simulink model "TUUM1_ME13"  (R2021b)
settings: Solver=ode1  StartTime=0.0  StopTime=Tsim  FixedStep=Ts  RelTol=1e-3
InitFcn:
  | Ts=1e-3;
  | Tsim=14.9;
  | TUUM1;
values from neighbouring files (symbols this model uses):
  REF = 5    [TUUM1.m]
undefined symbols (not defined in the file or in its folder): rtblkgui
libraries: simulink x3
settings Model: SimulationMode=external  Creator=Labos1  LastModifiedBy=Melab1Guest
settings SolverCC: AlgebraicLoopSolver=TrustRegion
settings DataIOCC: ReturnWorkspaceOutputs=off
settings OptimizationCC: LifeSpan=inf
settings DebuggingCC: SFExecutionAtInitializationDiag=none  SFMachineParentedDataDiag=warning  ArithmeticOperatorsInVariantConditions=warning
settings SFSimCC: SimUseLocalCustomCode=off  CustomCodeUndefinedFunction=UseInterfaceOnly
settings RTWCC: Description=Simulink Desktop Real-Time  SystemTargetFile=sldrt.tlc  TemplateMakefile=sldrt.tmf  RTWUseLocalCustomCode=off  RTWCompilerOptimization=on
settings CodeAppCC: MaxIdLength=95  StateflowObjectComments=on
settings SimulinkDesktopRealTimeCC: TargetPreCompLibLocation=C:\Program Files\MATLAB\R2021b\toolbox\sldrt\lib\win64  SupportVariableSizeSignals=off

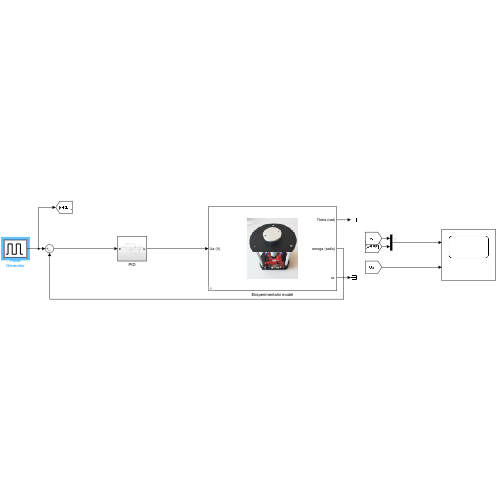
[thumbnail: Simulink's stored preview of the top-level diagram]
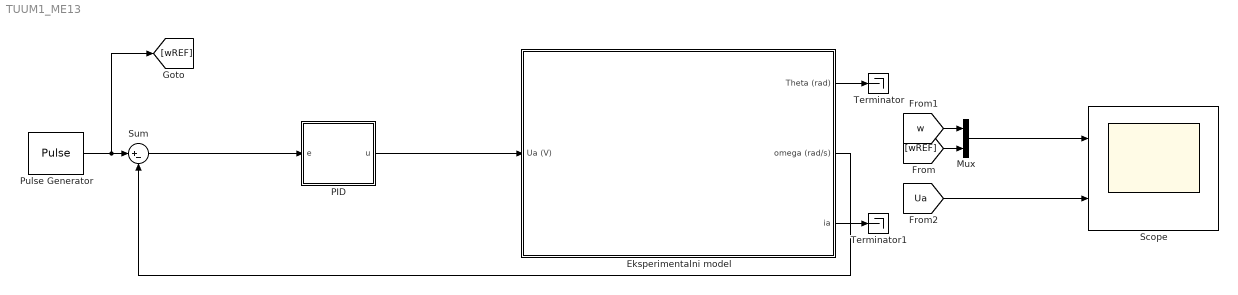
== system TUUM1_ME13 ==
  Eksperimentalni model : Subsystem  mask{R6=383, motorRes=2849.3, Ts=Ts}
      mask init:
      | currentBlock = gcb;
      | %% Closing all the ports:
      | Port = '';
      | FullPort = '';
      | if ~isempty(instrfind)
      |     fclose(instrfind);
      |     delete(instrfind);
      | end
      | %% Find all the COM ports in a computer
      | s1 = instrhwinfo('serial');
      | coms = s1.AvailableSerialPorts;
      | key = 'HKEY_LOCAL_MACHINE\SYSTEM\CurrentControlSet\Enum\USB\';
      | % Find all installed USB devices entries and clean up the output
      | [~, vals] = dos(['REG QUERY ' key ' /s /f "FriendlyName" /t "REG_SZ"']);
      | vals = textscan(vals,'%s','delimiter','\t');
      | vals = cat(1,vals{:});
      | out = 0;
      | % Find all friendly name property entries
      | for i = 1:numel(vals)
      |     if strcmp(vals{i}(1:min(12,end)),'FriendlyName')
      |         if ~iscell(out)
      |             out = vals(i);
      |         else
      |             out{end+1} = vals{i};
      |         end
      |     end
      | end
      | % Compare friendly name entries with connected ports and generate output
      | devs = cell(numel(coms),2);
      | for i = 1:numel(coms)
      |   match = strfind(out,[coms{i},')']);
      |   ind = 0;
      |   for j = 1:numel(match)
      |       if ~isempty(match{j})
      |           ind = j;
      |       end
      |   end
      |   if ind ~= 0
      |       com = str2double(coms{i}(4:end));
      | % Trim the trailing ' (COM##)' from the friendly name - works on ports from 1 to 99
      |       if com > 9
      |           length = 8;
      |       else
      |           length = 7;
      |       end
      |       devs{i,1} = out{ind}(27:end-length);
      |       devs{i,2} = com;
      |   end
      | end
      | % Find USB device
      | for i = size(devs,1)
      |     if strfind(devs{i,1},'USB Serial Device')
      |         ind = i;
      |     end
      | end
      | if ~ind
      |     Port = [];
      | else
      |     port = coms(ind);
      |     Port = port{1};
      | end
      | if (isempty(Port))
      |  %   msgbox('Barbell lab board not found, make sure it is connected, FTDI driver is installed and try again')
      | else
      |     %% Set Packet Input and Packet Output parameters
      |     po = strcat(currentBlock,'/Packet Output1');
      |     pinput = strcat(currentBlock,'/Packet Input1');
      |     %%
      |     set_param(po, 'LinkStatus','inactive');
      |     set_param(pinput, 'LinkStatus','inactive');
      |     %%
      |     p = Simulink.Mask.get(po);
      |     a = p.Parameters(6);
      |     FullPort = Port;
      |     Port = replace(Port,'COM','');
      |     if isempty(Port)
      |         Port = a.Value
      |     end
      |     %%
      | 
      |     a.set('Value',Port);
      |     %%
      |     %%
      |     %%
      |     p1 = Simulink.Mask.get(pinput);
      |     a1 = p1.Parameters(6);
      |     a1.set('Value',Port);
      | 
      | end
      mask Display:
      | ud = get_param(gcb,'UserData');
      | image(ud.x);
  Mux : Mux  Inputs=2
  PID : Subsystem
  Pulse Generator : DiscretePulseGenerator  PulseType=Time based  Amplitude=REF  Period=5  PulseWidth=50
  Scope : Scope  NumInputPorts=2
  Sum : Sum  Inputs=|+-
  Terminator : Terminator
  Terminator1 : Terminator
  wires:
  [w] -> Mux/1
  [wREF] -> Mux/2
  Pulse Generator/1 -> [wREF], Sum/1
  Eksperimentalni model/2(omega (rad/s)) -> Sum/2
  Mux/1 -> Scope/1
  [Ua] -> Scope/2
  Eksperimentalni model/1(Theta (rad)) -> Terminator/1
  Eksperimentalni model/3("ia ") -> Terminator1/1
  Sum/1 -> PID/1(e)
  PID/1(u) -> Eksperimentalni model/1(Ua (V))

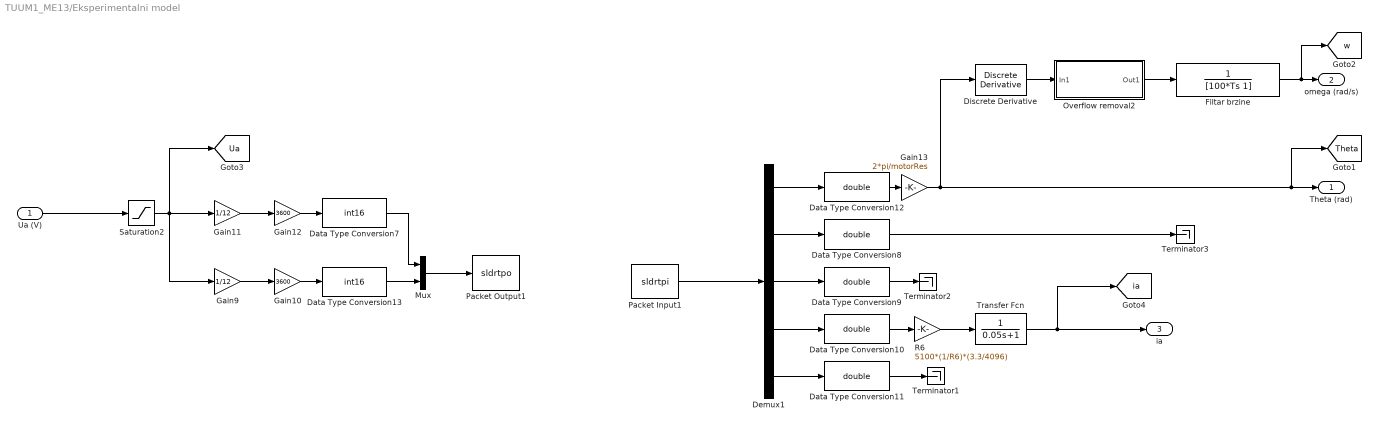
== system TUUM1_ME13/Eksperimentalni model ==
  Ua (V) : Inport
  Data Type Conversion{8..12} (5 alike) : DataTypeConversion  OutDataTypeStr=double
  Data Type Conversion13 : DataTypeConversion  OutDataTypeStr=int16
  Data Type Conversion7 : DataTypeConversion  OutDataTypeStr=int16
  Demux1 : Demux  Outputs=5
  Discrete Derivative : simulink/Discrete/Discrete Derivative  gainval=1.0  ICPrevScaledInput=0.0  OutMin=[]  OutMax=[]  OutDataType=fixdt(1, 16)  OutScaling=2^-10  DoSatur=off
  Filtar brzine : TransferFcn  Denominator=[100*Ts 1]
  Gain10 : Gain  Gain=3600
  Gain11 : Gain  Gain=1/12
  Gain12 : Gain  Gain=3600
  Gain13 : Gain  Gain=2*pi/motorRes  OutDataTypeStr=double
  Gain9 : Gain  Gain=1/12
  Mux : Mux  Inputs=2
  Overflow removal2 : Subsystem
  Packet Input1 : S-Function  LoadFcn=rtblkgui('Load')  StartFcn=rtblkgui('Start',1)  StopFcn=rtblkgui('Start',0)  FunctionName=sldrtpi  Parameters=SampleTime,MaxMissedTicks,ShowMissedTicks,YieldWhenWaiting,DrvName,DrvAddress,DrvOptions,PacketSize,DataTypes,ShowReady,ShowError,PacketID,ByteOrder,ShowTimestamp  SFunctionDeploymentMode=off  EnableBusSupport=off  mask(Simulink Desktop Real-Time Packet Input){SampleTime=Ts, MaxMissedTicks=10, ShowMissedTicks=off, YieldWhenWaiting=off, DrvName=Standard_Devices/Serial_Port, DrvAddress=9, DrvOptions=[115200 8 0 0 0 0 0 0], PacketSize=5*2, DataTypes='5*int16', ShowReady=off, ShowError=off, PacketID=1, ByteOrder=1, ShowTimestamp=off}
      mask prompts: SampleTime "sldrt:sldrtlib:ParamSampleTime"; MaxMissedTicks "sldrt:sldrtlib:ParamMaxMissedTicks"; ShowMissedTicks "sldrt:sldrtlib:ParamShowMissedTicks"; YieldWhenWaiting "sldrt:sldrtlib:ParamYieldWhenWaiting"; DrvName "sldrt:sldrtlib:ParamDriverName"; DrvAddress "sldrt:sldrtlib:ParamDriverAddress"; DrvOptions "sldrt:sldrtlib:ParamDriverOptions"; PacketSize "sldrt:sldrtlib:ParamInputPacketSize"; DataTypes "sldrt:sldrtlib:ParamPacketInputDataTypes"; ShowReady "sldrt:sldrtlib:ParamShowDataReady"; ShowError "sldrt:sldrtlib:ParamShowDataError"; PacketID "sldrt:sldrtlib:ParamPacketIdentifier"; ByteOrder "sldrt:sldrtlib:ParamPacketInputByteOrder"; ShowTimestamp "sldrt:sldrtlib:ParamShowPacketTimestamp"
      mask help: sldrt:sldrtlib:DescPacketInput
      settings: AttributesFormatString=Serial Port [3]  ModelCloseFcn=close(findall(0, 'Type', 'figure', 'Tag', 'SLDRT_RTBLKGUI', 'UserData', gcbh))  OpenFcn=rtblkgui('Open','PI')  ParentCloseFcn=eval(get_param(gcbh, 'ModelCloseFcn'))
      mask Help: helpview(fullfile(docroot, 'toolbox', 'sldrt', 'helptargets.map'), 'rtw_packet_in')
      mask Display: disp('Packet\nInput')
  Packet Output1 : S-Function  LoadFcn=rtblkgui('Load')  StartFcn=rtblkgui('Start',1)  StopFcn=rtblkgui('Start',0)  FunctionName=sldrtpo  Parameters=SampleTime,MaxMissedTicks,ShowMissedTicks,YieldWhenWaiting,DrvName,DrvAddress,DrvOptions,PacketSize,DataTypes,ShowReady,ShowError,PacketID,ByteOrder,InitialValue,FinalValue  SFunctionDeploymentMode=off  EnableBusSupport=off  mask(Simulink Desktop Real-Time Packet Output){SampleTime=Ts, MaxMissedTicks=10, ShowMissedTicks=off, YieldWhenWaiting=off, DrvName=Standard_Devices/Serial_Port, DrvAddress=9, DrvOptions=[115200 8 0 0 0 0 0 0], PacketSize=4, DataTypes='2*int16', ShowReady=off, ShowError=off, PacketID=1, ByteOrder=1, InitialValue=[32767 2], FinalValue=[0 0]}
      mask prompts: SampleTime "sldrt:sldrtlib:ParamSampleTime"; MaxMissedTicks "sldrt:sldrtlib:ParamMaxMissedTicks"; ShowMissedTicks "sldrt:sldrtlib:ParamShowMissedTicks"; YieldWhenWaiting "sldrt:sldrtlib:ParamYieldWhenWaiting"; DrvName "sldrt:sldrtlib:ParamDriverName"; DrvAddress "sldrt:sldrtlib:ParamDriverAddress"; DrvOptions "sldrt:sldrtlib:ParamDriverOptions"; PacketSize "sldrt:sldrtlib:ParamOutputPacketSize"; DataTypes "sldrt:sldrtlib:ParamPacketOutputDataTypes"; ShowReady "sldrt:sldrtlib:ParamShowDataReady"; ShowError "sldrt:sldrtlib:ParamShowDataError"; PacketID "sldrt:sldrtlib:ParamPacketIdentifier"; ByteOrder "sldrt:sldrtlib:ParamPacketOutputByteOrder"; InitialValue "sldrt:sldrtlib:ParamInitialValue"; FinalValue "sldrt:sldrtlib:ParamFinalValue"
      mask help: sldrt:sldrtlib:DescPacketOutput
      settings: AttributesFormatString=Serial Port [3]  ModelCloseFcn=close(findall(0, 'Type', 'figure', 'Tag', 'SLDRT_RTBLKGUI', 'UserData', gcbh))  OpenFcn=rtblkgui('Open','PO')  ParentCloseFcn=eval(get_param(gcbh, 'ModelCloseFcn'))
      mask Help: helpview(fullfile(docroot, 'toolbox', 'sldrt', 'helptargets.map'), 'rtw_packet_out')
      mask Display: disp('Packet\nOutput')
  R6 : Gain  Gain=5100*(1/R6)*(3.3/4096)
  Saturation2 : Saturate  UpperLimit=12  LowerLimit=-12
  Terminator1 : Terminator
  Terminator2 : Terminator
  Terminator3 : Terminator
  Transfer Fcn : TransferFcn  Denominator=[0.05 1]
  Theta (rad) : Outport  VectorParamsAs1DForOutWhenUnconnected=off
  omega (rad/s) : Outport  Port=2  VectorParamsAs1DForOutWhenUnconnected=off
  "ia " : Outport  Port=3  VectorParamsAs1DForOutWhenUnconnected=off
  tag scope: Theta=global, Ua=global, ia=global, w=global
  wires:
  Ua (V)/1 -> Saturation2/1
  Gain12/1 -> Data Type Conversion7/1
  Gain11/1 -> Gain12/1
  Gain10/1 -> Data Type Conversion13/1
  Gain9/1 -> Gain10/1
  Demux1/1 -> Data Type Conversion12/1
  Demux1/2 -> Data Type Conversion8/1
  Demux1/3 -> Data Type Conversion9/1
  Demux1/4 -> Data Type Conversion10/1
  Demux1/5 -> Data Type Conversion11/1
  Saturation2/1 -> [Ua], Gain9/1, Gain11/1
  Data Type Conversion7/1 -> Mux/1
  Data Type Conversion13/1 -> Mux/2
  Data Type Conversion8/1 -> Terminator3/1
  Data Type Conversion12/1 -> Gain13/1
  Gain13/1 -> [Theta], Theta (rad)/1, Discrete Derivative/1
  Discrete Derivative/1 -> Overflow removal2/1(In1)
  Filtar brzine/1 -> [w], omega (rad/s)/1
  Mux/1 -> Packet Output1/1
  Data Type Conversion11/1 -> Terminator1/1
  Data Type Conversion10/1 -> R6/1
  Data Type Conversion9/1 -> Terminator2/1
  R6/1 -> Transfer Fcn/1
  Overflow removal2/1(Out1) -> Filtar brzine/1
  Packet Input1/1 -> Demux1/1
  Transfer Fcn/1 -> [ia], "ia "/1

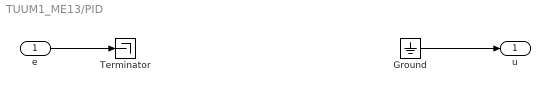
== system TUUM1_ME13/PID ==
  e : Inport
  Ground : Ground
  Terminator : Terminator
  u : Outport
  wires:
  e/1 -> Terminator/1
  Ground/1 -> u/1

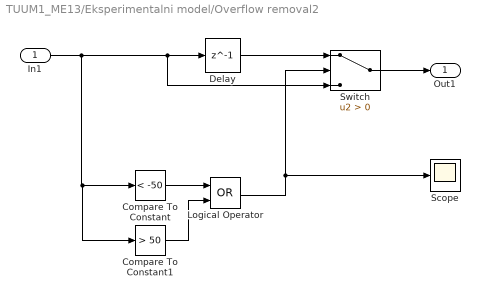
== system TUUM1_ME13/Eksperimentalni model/Overflow removal2 ==
  In1 : Inport
  Compare To Constant : simulink/Logic and Bit Operations/Compare To Constant  relop=<  const=-50  OutDataTypeStr=boolean
  Compare To Constant1 : simulink/Logic and Bit Operations/Compare To Constant  relop=>  const=50  OutDataTypeStr=boolean
  Delay : Delay  DelayLength=1  InitialCondition=0  UseCircularBuffer=on
  Logical Operator : Logic  Operator=OR  AllPortsSameDT=off  OutDataTypeStr=boolean
  Scope : Scope
  Switch : Switch  Criteria=u2 > Threshold
  Out1 : Outport  VectorParamsAs1DForOutWhenUnconnected=off
  wires:
  In1/1 -> Switch/3, Delay/1, Compare To Constant1/1, Compare To Constant/1
  Compare To Constant/1 -> Logical Operator/1
  Compare To Constant1/1 -> Logical Operator/2
  Delay/1 -> Switch/1
  Switch/1 -> Out1/1
  Logical Operator/1 -> Scope/1, Switch/2
